simulink model "SP_Dynamic_17Okt_ExergyFlow"  (R2019b)
settings: Solver=FixedStepAuto  StartTime=0.0  StopTime=0  FixedStep=1/3600  RelTol=1e-3
model workspace (MAT data in the model file):
  AD : Simulink.Parameter (value not decoded)
  AG : Simulink.Parameter (value not decoded)
  AH : Simulink.Parameter (value not decoded)
  AV : Simulink.Parameter (value not decoded)
  AVP : Simulink.Parameter (value not decoded)
  BCHL : Simulink.Parameter (value not decoded)
  BCHV : Simulink.Parameter (value not decoded)
  BD : Simulink.Parameter (value not decoded)
  BG : Simulink.Parameter (value not decoded)
  BH : Simulink.Parameter (value not decoded)
  BVP : Simulink.Parameter (value not decoded)
  CD : Simulink.Parameter (value not decoded)
  CG : Simulink.Parameter (value not decoded)
  CH : Simulink.Parameter (value not decoded)
  CVP : Simulink.Parameter (value not decoded)
  XMW : Simulink.Parameter (value not decoded)
symbols that are objects in the model workspace (value not decoded): AD, AG, AH, AV, AVP, BD, BG, BH, BVP, CD, CG, CH, CVP, XMW
undefined symbols (not defined in the file or in its folder): magnitude, SETPT, XMEAS, XMV
libraries: mylib x165, dspindex x17
(part 10 of 10)

== system SP_Dynamic_17Okt_ExergyFlow/Random number generator/Process Measurements XMEAS(I) I=1-22/If Action Subsystem3/Subsystem/Subsystem2/TESUB6 XMNS(12) ==
  G : Inport
  Process Noise I=1-12 G New : mylib/Process Noise I=1-12 G New  SystemSampleTime=-1  Latency=0  AutoFrameSizeCalculation=off
  XNS(12) : Constant  Value=1.0000
  XMNS : Outport  VectorParamsAs1DForOutWhenUnconnected=off
  G_NEW : Outport  Port=2  VectorParamsAs1DForOutWhenUnconnected=off
  wires:
  XNS(12)/1 -> Process Noise I=1-12 G New/1
  Process Noise I=1-12 G New/1 -> XMNS/1
  G/1 -> Process Noise I=1-12 G New/2
  Process Noise I=1-12 G New/2 -> G_NEW/1

== system SP_Dynamic_17Okt_ExergyFlow/Random number generator/Process Measurements XMEAS(I) I=1-22/If Action Subsystem3/Subsystem/Subsystem2/TESUB6 XMNS(13) ==
  G : Inport
  Process Noise I=1-12 G New : mylib/Process Noise I=1-12 G New  SystemSampleTime=-1  Latency=0  AutoFrameSizeCalculation=off
  XNS(13) : Constant  Value=0.3000
  XMNS : Outport  VectorParamsAs1DForOutWhenUnconnected=off
  G_NEW : Outport  Port=2  VectorParamsAs1DForOutWhenUnconnected=off
  wires:
  XNS(13)/1 -> Process Noise I=1-12 G New/1
  Process Noise I=1-12 G New/1 -> XMNS/1
  G/1 -> Process Noise I=1-12 G New/2
  Process Noise I=1-12 G New/2 -> G_NEW/1

== system SP_Dynamic_17Okt_ExergyFlow/Random number generator/Process Measurements XMEAS(I) I=1-22/If Action Subsystem3/Subsystem/Subsystem2/TESUB6 XMNS(14) ==
  G : Inport
  Process Noise I=1-12 G New : mylib/Process Noise I=1-12 G New  SystemSampleTime=-1  Latency=0  AutoFrameSizeCalculation=off
  XNS(14) : Constant  Value=0.1250
  XMNS : Outport  VectorParamsAs1DForOutWhenUnconnected=off
  G_NEW : Outport  Port=2  VectorParamsAs1DForOutWhenUnconnected=off
  wires:
  XNS(14)/1 -> Process Noise I=1-12 G New/1
  Process Noise I=1-12 G New/1 -> XMNS/1
  G/1 -> Process Noise I=1-12 G New/2
  Process Noise I=1-12 G New/2 -> G_NEW/1

== system SP_Dynamic_17Okt_ExergyFlow/Random number generator/Process Measurements XMEAS(I) I=1-22/If Action Subsystem3/Subsystem/Subsystem2/TESUB6 XMNS(15) ==
  G : Inport
  Process Noise I=1-12 G New : mylib/Process Noise I=1-12 G New  SystemSampleTime=-1  Latency=0  AutoFrameSizeCalculation=off
  XNS(15) : Constant  Value=1.0000
  XMNS : Outport  VectorParamsAs1DForOutWhenUnconnected=off
  G_NEW : Outport  Port=2  VectorParamsAs1DForOutWhenUnconnected=off
  wires:
  XNS(15)/1 -> Process Noise I=1-12 G New/1
  Process Noise I=1-12 G New/1 -> XMNS/1
  G/1 -> Process Noise I=1-12 G New/2
  Process Noise I=1-12 G New/2 -> G_NEW/1

== system SP_Dynamic_17Okt_ExergyFlow/Random number generator/Process Measurements XMEAS(I) I=1-22/If Action Subsystem3/Subsystem/Subsystem3/TESUB6 XMNS(16) ==
  G : Inport
  Process Noise I=1-12 G New : mylib/Process Noise I=1-12 G New  SystemSampleTime=-1  Latency=0  AutoFrameSizeCalculation=off
  XNS(16) : Constant  Value=0.3000
  XMNS : Outport  VectorParamsAs1DForOutWhenUnconnected=off
  G_NEW : Outport  Port=2  VectorParamsAs1DForOutWhenUnconnected=off
  wires:
  XNS(16)/1 -> Process Noise I=1-12 G New/1
  Process Noise I=1-12 G New/1 -> XMNS/1
  G/1 -> Process Noise I=1-12 G New/2
  Process Noise I=1-12 G New/2 -> G_NEW/1

== system SP_Dynamic_17Okt_ExergyFlow/Random number generator/Process Measurements XMEAS(I) I=1-22/If Action Subsystem3/Subsystem/Subsystem3/TESUB6 XMNS(17) ==
  G : Inport
  Process Noise I=1-12 G New : mylib/Process Noise I=1-12 G New  SystemSampleTime=-1  Latency=0  AutoFrameSizeCalculation=off
  XNS(17) : Constant  Value=0.1150
  XMNS : Outport  VectorParamsAs1DForOutWhenUnconnected=off
  G_NEW : Outport  Port=2  VectorParamsAs1DForOutWhenUnconnected=off
  wires:
  XNS(17)/1 -> Process Noise I=1-12 G New/1
  Process Noise I=1-12 G New/1 -> XMNS/1
  G/1 -> Process Noise I=1-12 G New/2
  Process Noise I=1-12 G New/2 -> G_NEW/1

== system SP_Dynamic_17Okt_ExergyFlow/Random number generator/Process Measurements XMEAS(I) I=1-22/If Action Subsystem3/Subsystem/Subsystem3/TESUB6 XMNS(18) ==
  G : Inport
  Process Noise I=1-12 G New : mylib/Process Noise I=1-12 G New  SystemSampleTime=-1  Latency=0  AutoFrameSizeCalculation=off
  XNS(18) : Constant  Value=0.0100
  XMNS : Outport  VectorParamsAs1DForOutWhenUnconnected=off
  G_NEW : Outport  Port=2  VectorParamsAs1DForOutWhenUnconnected=off
  wires:
  XNS(18)/1 -> Process Noise I=1-12 G New/1
  Process Noise I=1-12 G New/1 -> XMNS/1
  G/1 -> Process Noise I=1-12 G New/2
  Process Noise I=1-12 G New/2 -> G_NEW/1

== system SP_Dynamic_17Okt_ExergyFlow/Random number generator/Process Measurements XMEAS(I) I=1-22/If Action Subsystem3/Subsystem/Subsystem3/TESUB6 XMNS(19) ==
  G : Inport
  Process Noise I=1-12 G New : mylib/Process Noise I=1-12 G New  SystemSampleTime=-1  Latency=0  AutoFrameSizeCalculation=off
  XNS(19) : Constant  Value=1.1500
  XMNS : Outport  VectorParamsAs1DForOutWhenUnconnected=off
  G_NEW : Outport  Port=2  VectorParamsAs1DForOutWhenUnconnected=off
  wires:
  XNS(19)/1 -> Process Noise I=1-12 G New/1
  Process Noise I=1-12 G New/1 -> XMNS/1
  G/1 -> Process Noise I=1-12 G New/2
  Process Noise I=1-12 G New/2 -> G_NEW/1

== system SP_Dynamic_17Okt_ExergyFlow/Random number generator/Process Measurements XMEAS(I) I=1-22/If Action Subsystem3/Subsystem/Subsystem3/TESUB6 XMNS(20) ==
  G : Inport
  Process Noise I=1-12 G New : mylib/Process Noise I=1-12 G New  SystemSampleTime=-1  Latency=0  AutoFrameSizeCalculation=off
  XNS(20) : Constant  Value=0.2000
  XMNS : Outport  VectorParamsAs1DForOutWhenUnconnected=off
  G_NEW : Outport  Port=2  VectorParamsAs1DForOutWhenUnconnected=off
  wires:
  XNS(20)/1 -> Process Noise I=1-12 G New/1
  Process Noise I=1-12 G New/1 -> XMNS/1
  G/1 -> Process Noise I=1-12 G New/2
  Process Noise I=1-12 G New/2 -> G_NEW/1

== system SP_Dynamic_17Okt_ExergyFlow/Random number generator/Process Measurements XMEAS(I) I=1-22/If Action Subsystem3/Subsystem/Subsystem3/TESUB6 XMNS(21) ==
  G : Inport
  Process Noise I=1-12 G New : mylib/Process Noise I=1-12 G New  SystemSampleTime=-1  Latency=0  AutoFrameSizeCalculation=off
  XNS(21) : Constant  Value=0.0100
  XMNS : Outport  VectorParamsAs1DForOutWhenUnconnected=off
  G_NEW : Outport  Port=2  VectorParamsAs1DForOutWhenUnconnected=off
  wires:
  XNS(21)/1 -> Process Noise I=1-12 G New/1
  Process Noise I=1-12 G New/1 -> XMNS/1
  G/1 -> Process Noise I=1-12 G New/2
  Process Noise I=1-12 G New/2 -> G_NEW/1

== system SP_Dynamic_17Okt_ExergyFlow/Random number generator/Process Measurements XMEAS(I) I=1-22/If Action Subsystem3/Subsystem/Subsystem3/TESUB6 XMNS(22) ==
  G : Inport
  Process Noise I=1-12 G New : mylib/Process Noise I=1-12 G New  SystemSampleTime=-1  Latency=0  AutoFrameSizeCalculation=off
  XNS(22) : Constant  Value=0.0100
  XMNS : Outport  VectorParamsAs1DForOutWhenUnconnected=off
  G_NEW : Outport  Port=2  VectorParamsAs1DForOutWhenUnconnected=off
  wires:
  XNS(22)/1 -> Process Noise I=1-12 G New/1
  Process Noise I=1-12 G New/1 -> XMNS/1
  G/1 -> Process Noise I=1-12 G New/2
  Process Noise I=1-12 G New/2 -> G_NEW/1

== system SP_Dynamic_17Okt_ExergyFlow/Random number generator/Process Measurements XMEAS(I) I=23-36/If Action Subsystem3/Subsystem/Subsystem/TESUB6 XMNS(23) ==
  G : Inport
  Process Noise I=1-12 G New : mylib/Process Noise I=1-12 G New  SystemSampleTime=-1  Latency=0  AutoFrameSizeCalculation=off
  XNS(23) : Constant  Value=0.25
  XMNS : Outport  VectorParamsAs1DForOutWhenUnconnected=off
  G_NEW : Outport  Port=2  VectorParamsAs1DForOutWhenUnconnected=off
  wires:
  XNS(23)/1 -> Process Noise I=1-12 G New/1
  Process Noise I=1-12 G New/1 -> XMNS/1
  G/1 -> Process Noise I=1-12 G New/2
  Process Noise I=1-12 G New/2 -> G_NEW/1

== system SP_Dynamic_17Okt_ExergyFlow/Random number generator/Process Measurements XMEAS(I) I=23-36/If Action Subsystem3/Subsystem/Subsystem/TESUB6 XMNS(24) ==
  G : Inport
  Process Noise I=1-12 G New : mylib/Process Noise I=1-12 G New  SystemSampleTime=-1  Latency=0  AutoFrameSizeCalculation=off
  XNS(24) : Constant  Value=0.1
  XMNS : Outport  VectorParamsAs1DForOutWhenUnconnected=off
  G_NEW : Outport  Port=2  VectorParamsAs1DForOutWhenUnconnected=off
  wires:
  XNS(24)/1 -> Process Noise I=1-12 G New/1
  Process Noise I=1-12 G New/1 -> XMNS/1
  G/1 -> Process Noise I=1-12 G New/2
  Process Noise I=1-12 G New/2 -> G_NEW/1

== system SP_Dynamic_17Okt_ExergyFlow/Random number generator/Process Measurements XMEAS(I) I=23-36/If Action Subsystem3/Subsystem/Subsystem/TESUB6 XMNS(25) ==
  G : Inport
  Process Noise I=1-12 G New : mylib/Process Noise I=1-12 G New  SystemSampleTime=-1  Latency=0  AutoFrameSizeCalculation=off
  XNS(25) : Constant  Value=0.25
  XMNS : Outport  VectorParamsAs1DForOutWhenUnconnected=off
  G_NEW : Outport  Port=2  VectorParamsAs1DForOutWhenUnconnected=off
  wires:
  XNS(25)/1 -> Process Noise I=1-12 G New/1
  Process Noise I=1-12 G New/1 -> XMNS/1
  G/1 -> Process Noise I=1-12 G New/2
  Process Noise I=1-12 G New/2 -> G_NEW/1

== system SP_Dynamic_17Okt_ExergyFlow/Random number generator/Process Measurements XMEAS(I) I=23-36/If Action Subsystem3/Subsystem/Subsystem/TESUB6 XMNS(26) ==
  G : Inport
  Process Noise I=1-12 G New : mylib/Process Noise I=1-12 G New  SystemSampleTime=-1  Latency=0  AutoFrameSizeCalculation=off
  XNS(26) : Constant  Value=0.1
  XMNS : Outport  VectorParamsAs1DForOutWhenUnconnected=off
  G_NEW : Outport  Port=2  VectorParamsAs1DForOutWhenUnconnected=off
  wires:
  XNS(26)/1 -> Process Noise I=1-12 G New/1
  Process Noise I=1-12 G New/1 -> XMNS/1
  G/1 -> Process Noise I=1-12 G New/2
  Process Noise I=1-12 G New/2 -> G_NEW/1

== system SP_Dynamic_17Okt_ExergyFlow/Random number generator/Process Measurements XMEAS(I) I=23-36/If Action Subsystem3/Subsystem/Subsystem/TESUB6 XMNS(27) ==
  G : Inport
  Process Noise I=1-12 G New : mylib/Process Noise I=1-12 G New  SystemSampleTime=-1  Latency=0  AutoFrameSizeCalculation=off
  XNS(27) : Constant  Value=0.25
  XMNS : Outport  VectorParamsAs1DForOutWhenUnconnected=off
  G_NEW : Outport  Port=2  VectorParamsAs1DForOutWhenUnconnected=off
  wires:
  XNS(27)/1 -> Process Noise I=1-12 G New/1
  Process Noise I=1-12 G New/1 -> XMNS/1
  G/1 -> Process Noise I=1-12 G New/2
  Process Noise I=1-12 G New/2 -> G_NEW/1

== system SP_Dynamic_17Okt_ExergyFlow/Random number generator/Process Measurements XMEAS(I) I=23-36/If Action Subsystem3/Subsystem/Subsystem1/TESUB6 XMNS(28) ==
  G : Inport
  Process Noise I=1-12 G New : mylib/Process Noise I=1-12 G New  SystemSampleTime=-1  Latency=0  AutoFrameSizeCalculation=off
  XNS(28) : Constant  Value=0.025
  XMNS : Outport  VectorParamsAs1DForOutWhenUnconnected=off
  G_NEW : Outport  Port=2  VectorParamsAs1DForOutWhenUnconnected=off
  wires:
  XNS(28)/1 -> Process Noise I=1-12 G New/1
  Process Noise I=1-12 G New/1 -> XMNS/1
  G/1 -> Process Noise I=1-12 G New/2
  Process Noise I=1-12 G New/2 -> G_NEW/1

== system SP_Dynamic_17Okt_ExergyFlow/Random number generator/Process Measurements XMEAS(I) I=23-36/If Action Subsystem3/Subsystem/Subsystem1/TESUB6 XMNS(29) ==
  G : Inport
  Process Noise I=1-12 G New : mylib/Process Noise I=1-12 G New  SystemSampleTime=-1  Latency=0  AutoFrameSizeCalculation=off
  XNS(29) : Constant  Value=0.25
  XMNS : Outport  VectorParamsAs1DForOutWhenUnconnected=off
  G_NEW : Outport  Port=2  VectorParamsAs1DForOutWhenUnconnected=off
  wires:
  XNS(29)/1 -> Process Noise I=1-12 G New/1
  Process Noise I=1-12 G New/1 -> XMNS/1
  G/1 -> Process Noise I=1-12 G New/2
  Process Noise I=1-12 G New/2 -> G_NEW/1

== system SP_Dynamic_17Okt_ExergyFlow/Random number generator/Process Measurements XMEAS(I) I=23-36/If Action Subsystem3/Subsystem/Subsystem1/TESUB6 XMNS(30) ==
  G : Inport
  Process Noise I=1-12 G New : mylib/Process Noise I=1-12 G New  SystemSampleTime=-1  Latency=0  AutoFrameSizeCalculation=off
  XNS(30) : Constant  Value=0.1
  XMNS : Outport  VectorParamsAs1DForOutWhenUnconnected=off
  G_NEW : Outport  Port=2  VectorParamsAs1DForOutWhenUnconnected=off
  wires:
  XNS(30)/1 -> Process Noise I=1-12 G New/1
  Process Noise I=1-12 G New/1 -> XMNS/1
  G/1 -> Process Noise I=1-12 G New/2
  Process Noise I=1-12 G New/2 -> G_NEW/1

== system SP_Dynamic_17Okt_ExergyFlow/Random number generator/Process Measurements XMEAS(I) I=23-36/If Action Subsystem3/Subsystem/Subsystem1/TESUB6 XMNS(31) ==
  G : Inport
  Process Noise I=1-12 G New : mylib/Process Noise I=1-12 G New  SystemSampleTime=-1  Latency=0  AutoFrameSizeCalculation=off
  XNS(31) : Constant  Value=0.25
  XMNS : Outport  VectorParamsAs1DForOutWhenUnconnected=off
  G_NEW : Outport  Port=2  VectorParamsAs1DForOutWhenUnconnected=off
  wires:
  XNS(31)/1 -> Process Noise I=1-12 G New/1
  Process Noise I=1-12 G New/1 -> XMNS/1
  G/1 -> Process Noise I=1-12 G New/2
  Process Noise I=1-12 G New/2 -> G_NEW/1

== system SP_Dynamic_17Okt_ExergyFlow/Random number generator/Process Measurements XMEAS(I) I=23-36/If Action Subsystem3/Subsystem/Subsystem1/TESUB6 XMNS(32) ==
  G : Inport
  Process Noise I=1-12 G New : mylib/Process Noise I=1-12 G New  SystemSampleTime=-1  Latency=0  AutoFrameSizeCalculation=off
  XNS(32) : Constant  Value=0.1
  XMNS : Outport  VectorParamsAs1DForOutWhenUnconnected=off
  G_NEW : Outport  Port=2  VectorParamsAs1DForOutWhenUnconnected=off
  wires:
  XNS(32)/1 -> Process Noise I=1-12 G New/1
  Process Noise I=1-12 G New/1 -> XMNS/1
  G/1 -> Process Noise I=1-12 G New/2
  Process Noise I=1-12 G New/2 -> G_NEW/1

== system SP_Dynamic_17Okt_ExergyFlow/Random number generator/Process Measurements XMEAS(I) I=23-36/If Action Subsystem3/Subsystem/Subsystem2/TESUB6 XMNS(33) ==
  G : Inport
  Process Noise I=1-12 G New : mylib/Process Noise I=1-12 G New  SystemSampleTime=-1  Latency=0  AutoFrameSizeCalculation=off
  XNS(33) : Constant  Value=0.25
  XMNS : Outport  VectorParamsAs1DForOutWhenUnconnected=off
  G_NEW : Outport  Port=2  VectorParamsAs1DForOutWhenUnconnected=off
  wires:
  XNS(33)/1 -> Process Noise I=1-12 G New/1
  Process Noise I=1-12 G New/1 -> XMNS/1
  G/1 -> Process Noise I=1-12 G New/2
  Process Noise I=1-12 G New/2 -> G_NEW/1

== system SP_Dynamic_17Okt_ExergyFlow/Random number generator/Process Measurements XMEAS(I) I=23-36/If Action Subsystem3/Subsystem/Subsystem2/TESUB6 XMNS(34) ==
  G : Inport
  Process Noise I=1-12 G New : mylib/Process Noise I=1-12 G New  SystemSampleTime=-1  Latency=0  AutoFrameSizeCalculation=off
  XNS(34) : Constant  Value=0.025
  XMNS : Outport  VectorParamsAs1DForOutWhenUnconnected=off
  G_NEW : Outport  Port=2  VectorParamsAs1DForOutWhenUnconnected=off
  wires:
  XNS(34)/1 -> Process Noise I=1-12 G New/1
  Process Noise I=1-12 G New/1 -> XMNS/1
  G/1 -> Process Noise I=1-12 G New/2
  Process Noise I=1-12 G New/2 -> G_NEW/1

== system SP_Dynamic_17Okt_ExergyFlow/Random number generator/Process Measurements XMEAS(I) I=23-36/If Action Subsystem3/Subsystem/Subsystem2/TESUB6 XMNS(35) ==
  G : Inport
  Process Noise I=1-12 G New : mylib/Process Noise I=1-12 G New  SystemSampleTime=-1  Latency=0  AutoFrameSizeCalculation=off
  XNS(35) : Constant  Value=0.05
  XMNS : Outport  VectorParamsAs1DForOutWhenUnconnected=off
  G_NEW : Outport  Port=2  VectorParamsAs1DForOutWhenUnconnected=off
  wires:
  XNS(35)/1 -> Process Noise I=1-12 G New/1
  Process Noise I=1-12 G New/1 -> XMNS/1
  G/1 -> Process Noise I=1-12 G New/2
  Process Noise I=1-12 G New/2 -> G_NEW/1

== system SP_Dynamic_17Okt_ExergyFlow/Random number generator/Process Measurements XMEAS(I) I=23-36/If Action Subsystem3/Subsystem/Subsystem2/TESUB6 XMNS(36) ==
  G : Inport
  Process Noise I=1-12 G New : mylib/Process Noise I=1-12 G New  SystemSampleTime=-1  Latency=0  AutoFrameSizeCalculation=off
  XNS(36) : Constant  Value=0.05
  XMNS : Outport  VectorParamsAs1DForOutWhenUnconnected=off
  G_NEW : Outport  Port=2  VectorParamsAs1DForOutWhenUnconnected=off
  wires:
  XNS(36)/1 -> Process Noise I=1-12 G New/1
  Process Noise I=1-12 G New/1 -> XMNS/1
  G/1 -> Process Noise I=1-12 G New/2
  Process Noise I=1-12 G New/2 -> G_NEW/1

== system SP_Dynamic_17Okt_ExergyFlow/Random number generator/Process Measurements XMEAS(I) I=37-41/If Action Subsystem3/Subsystem/Subsystem/TESUB6 XMNS(37) ==
  G : Inport
  Process Noise I=1-12 G New : mylib/Process Noise I=1-12 G New  SystemSampleTime=-1  Latency=0  AutoFrameSizeCalculation=off
  XNS(37) : Constant  Value=0.01
  XMNS : Outport  VectorParamsAs1DForOutWhenUnconnected=off
  G_NEW : Outport  Port=2  VectorParamsAs1DForOutWhenUnconnected=off
  wires:
  XNS(37)/1 -> Process Noise I=1-12 G New/1
  Process Noise I=1-12 G New/1 -> XMNS/1
  G/1 -> Process Noise I=1-12 G New/2
  Process Noise I=1-12 G New/2 -> G_NEW/1

== system SP_Dynamic_17Okt_ExergyFlow/Random number generator/Process Measurements XMEAS(I) I=37-41/If Action Subsystem3/Subsystem/Subsystem/TESUB6 XMNS(38) ==
  G : Inport
  Process Noise I=1-12 G New : mylib/Process Noise I=1-12 G New  SystemSampleTime=-1  Latency=0  AutoFrameSizeCalculation=off
  XNS(38) : Constant  Value=0.01
  XMNS : Outport  VectorParamsAs1DForOutWhenUnconnected=off
  G_NEW : Outport  Port=2  VectorParamsAs1DForOutWhenUnconnected=off
  wires:
  XNS(38)/1 -> Process Noise I=1-12 G New/1
  Process Noise I=1-12 G New/1 -> XMNS/1
  G/1 -> Process Noise I=1-12 G New/2
  Process Noise I=1-12 G New/2 -> G_NEW/1

== system SP_Dynamic_17Okt_ExergyFlow/Random number generator/Process Measurements XMEAS(I) I=37-41/If Action Subsystem3/Subsystem/Subsystem/TESUB6 XMNS(39) ==
  G : Inport
  Process Noise I=1-12 G New : mylib/Process Noise I=1-12 G New  SystemSampleTime=-1  Latency=0  AutoFrameSizeCalculation=off
  XNS(39) : Constant  Value=0.01
  XMNS : Outport  VectorParamsAs1DForOutWhenUnconnected=off
  G_NEW : Outport  Port=2  VectorParamsAs1DForOutWhenUnconnected=off
  wires:
  XNS(39)/1 -> Process Noise I=1-12 G New/1
  Process Noise I=1-12 G New/1 -> XMNS/1
  G/1 -> Process Noise I=1-12 G New/2
  Process Noise I=1-12 G New/2 -> G_NEW/1

== system SP_Dynamic_17Okt_ExergyFlow/Random number generator/Process Measurements XMEAS(I) I=37-41/If Action Subsystem3/Subsystem/Subsystem/TESUB6 XMNS(40) ==
  G : Inport
  Process Noise I=1-12 G New : mylib/Process Noise I=1-12 G New  SystemSampleTime=-1  Latency=0  AutoFrameSizeCalculation=off
  XNS(40) : Constant  Value=0.5
  XMNS : Outport  VectorParamsAs1DForOutWhenUnconnected=off
  G_NEW : Outport  Port=2  VectorParamsAs1DForOutWhenUnconnected=off
  wires:
  XNS(40)/1 -> Process Noise I=1-12 G New/1
  Process Noise I=1-12 G New/1 -> XMNS/1
  G/1 -> Process Noise I=1-12 G New/2
  Process Noise I=1-12 G New/2 -> G_NEW/1

== system SP_Dynamic_17Okt_ExergyFlow/Random number generator/Process Measurements XMEAS(I) I=37-41/If Action Subsystem3/Subsystem/Subsystem/TESUB6 XMNS(41) ==
  G : Inport
  Process Noise I=1-12 G New : mylib/Process Noise I=1-12 G New  SystemSampleTime=-1  Latency=0  AutoFrameSizeCalculation=off
  XNS(41) : Constant  Value=0.5
  XMNS : Outport  VectorParamsAs1DForOutWhenUnconnected=off
  G_NEW : Outport  Port=2  VectorParamsAs1DForOutWhenUnconnected=off
  wires:
  XNS(41)/1 -> Process Noise I=1-12 G New/1
  Process Noise I=1-12 G New/1 -> XMNS/1
  G/1 -> Process Noise I=1-12 G New/2
  Process Noise I=1-12 G New/2 -> G_NEW/1

== system SP_Dynamic_17Okt_ExergyFlow/Subsystem/Braatz/ 10/CONTROL 6/P Control/ERR ==
  SETPT : Inport
  High Limit : Inport  Port=2
  XMEAS : Inport  Port=3
  " " : Product  Inputs=**/
  Bus Selector : BusSelector  OutputSignals=signal3.XMEAS(10)
  Constant : Constant  Value=100
  Subtract : Sum  Inputs=+-
  ERR : Outport  VectorParamsAs1DForOutWhenUnconnected=off
  wires:
  " "/1 -> ERR/1
  SETPT/1 -> Subtract/1
  Subtract/1 -> " "/1
  High Limit/1 -> " "/3
  Constant/1 -> " "/2
  XMEAS/1 -> Bus Selector/1
  Bus Selector/1 -> Subtract/2  "<XMEAS(10)>"

== system SP_Dynamic_17Okt_ExergyFlow/Subsystem/Braatz/ 10/CONTROL 6/P Control/Pressure limits ==
  "XMV(6) " : Inport
  XMEAS : Inport  Port=2
  Abs : Abs
  Bus Selector : BusSelector  OutputSignals=signal3.XMEAS(13)
  Constant : Constant  Value=100
  Constant1 : Constant  Value=0
  If : If  IfExpression=u1 >= 2950  ElseIfExpressions=u1 <= 2300
  If Action Subsystem : Subsystem  TreatAsAtomicUnit=on
  If Action Subsystem1 : Subsystem  TreatAsAtomicUnit=on
  If Action Subsystem2 : Subsystem  TreatAsAtomicUnit=on
  Merge : Merge  Inputs=3
  Subsystem1 : mylib/Braatz Control/Subsystem1  SystemSampleTime=-1  Latency=0  AutoFrameSizeCalculation=off
  XMV(6) : Outport  VectorParamsAs1DForOutWhenUnconnected=off
  wires:
  If/1 -> If Action Subsystem/Action
  Constant1/1 -> If Action Subsystem1/1(In1)
  Merge/1 -> Abs/1
  If/3 -> If Action Subsystem2/Action
  Constant/1 -> If Action Subsystem/1(In1)
  Bus Selector/1 -> If/1  "<XMEAS(13)>"
  If Action Subsystem2/1(Out1) -> Merge/3
  If Action Subsystem1/1(Out1) -> Merge/2
  XMEAS/1 -> Bus Selector/1
  If/2 -> If Action Subsystem1/Action
  If Action Subsystem/1(Out1) -> Merge/1
  "XMV(6) "/1 -> If Action Subsystem2/1(In1)
  Abs/1 -> Subsystem1/1
  Subsystem1/1 -> XMV(6)/1

== system SP_Dynamic_17Okt_ExergyFlow/Subsystem/Braatz/ 10/CONTROL 6/P Control/Subsystem ==
  ERR : Inport
  GAIN : Inport  Port=2
  ERROLD : UnitDelay  SampleTime=-1  HasFrameUpgradeWarning=on
  Product : Product
  Subtract1 : Sum  Inputs=+-
  DXMV : Outport  VectorParamsAs1DForOutWhenUnconnected=off
  wires:
  ERR/1 -> Subtract1/1, ERROLD/1
  ERROLD/1 -> Subtract1/2
  Subtract1/1 -> Product/2
  Product/1 -> DXMV/1
  GAIN/1 -> Product/1

== system SP_Dynamic_17Okt_ExergyFlow/Subsystem/Braatz/ 10/CONTROL 6/P Control/Pressure limits/If Action Subsystem ==
  In1 : Inport
  Action Port : ActionPort  ActionPortLabel=if(u1 >= 2950)
  Out1 : Outport  VectorParamsAs1DForOutWhenUnconnected=off
  wires:
  In1/1 -> Out1/1

== system SP_Dynamic_17Okt_ExergyFlow/Subsystem/Braatz/ 10/CONTROL 6/P Control/Pressure limits/If Action Subsystem1 ==
  In1 : Inport
  Action Port : ActionPort  ActionPortLabel=elseif(u1 <= 2300)
  Out1 : Outport  VectorParamsAs1DForOutWhenUnconnected=off
  wires:
  In1/1 -> Out1/1

== system SP_Dynamic_17Okt_ExergyFlow/Subsystem/Braatz/ 10/CONTROL 6/P Control/Pressure limits/If Action Subsystem2 ==
  In1 : Inport
  Action Port : ActionPort  ActionPortLabel=else
  Out1 : Outport  VectorParamsAs1DForOutWhenUnconnected=off
  wires:
  In1/1 -> Out1/1

== matlab function SP_Dynamic_17Okt_ExergyFlow/Separator/TCS Initial Temperature in Separator °C /MATLAB Function ==
  data: AH input; TCS output; BH input; CH input; AG input; BG input; CG input; AV input; XMW input; XLS input; ETS input; UTLS input; ITY input; J output; TCS input
function [TCS,J] = TempLoop(AH,BH,CH,AG,BG,CG,AV,XMW,XLS,ETS,UTLS,ITY,TCS)

ESS = ETS/UTLS;
     
Z = XLS;
T = TCS;
H = ESS;
TIN=T;

for J = 1:100
	
	if ITY == 0
    	HTEST = 0;
		for I = 1:8
      		HI = T * (AH(I,1) + BH(I,1) * T / 2 + CH(I,1) * T^2 / 3);
      		HI = 1.8 * HI;
      		HTEST = HTEST + Z(I,1) * XMW(I,1) * HI;
		end
	else
      	HTEST = 0;
		for I = 1:8 
      		HI = T * (AG(I,1) + BG(I,1) * T / 2 + CG(I,1) * T^2 / 3);
      		HI = 1.8 * HI;
      		HI = HI + AV(I,1);
      		HTEST = HTEST + Z(I,1) * XMW(I,1) * HI;
		end
    end
        if ITY == 2
         	R1 = 3.57696 / 1000000;
        	HTEST = HTEST - R1 * (T + 273.15);
    	end
		
    ERR = HTEST - H;
	
	if ITY == 0
      	DH = 0.0;
    	for I = 1:8
      		DHI = AH(I,1) + BH(I,1) * T + CH(I,1) * T^2;
      		DHI = 1.8 * DHI;
      		DH = DH + Z(I,1) * XMW(I,1) * DHI;
		end
	else
      	DH=0.0;
    	for I = 1:8
      		DHI = AG(I,1) + BG(I,1) * T + CG(I,1) * T^2;
      		DHI = 1.8 * DHI;
      		DH = DH + Z(I,1) * XMW(I,1) * DHI;
		end
    end
    
    if ITY == 2
      	R3 = 3.57696/1000000;
     	DH = DH - R3;
 	end
	
    DT = -ERR / DH;
    T = T + DT;
  	if abs(DT) < 1*10^(-12)
    	break
  	end
  	if J == 100
  		T = TIN;
  	end
end
TCS = T;

== matlab function SP_Dynamic_17Okt_ExergyFlow/Reactor/TCR Initial Temperature in Reactor °C /MATLAB Function ==
  data: AH input; TCR output; BH input; CH input; AG input; BG input; CG input; AV input; XMW input; XLR input; ETR input; UTLR input; ITY input; J output; TCR input
function [TCR,J] = TempLoop(AH,BH,CH,AG,BG,CG,AV,XMW,XLR,ETR,UTLR,ITY,TCR)

ESR = ETR/UTLR;
     
Z = XLR;
T = TCR;
H = ESR;
TIN=T;

for J = 1:100
	
	if ITY == 0
    	HTEST = 0;
		for I = 1:8
      		HI = T * (AH(I,1) + BH(I,1) * T / 2 + CH(I,1) * T^2 / 3);
      		HI = 1.8 * HI;
      		HTEST = HTEST + Z(I,1) * XMW(I,1) * HI;
		end
	else
      	HTEST = 0;
		for I = 1:8 
      		HI = T * (AG(I,1) + BG(I,1) * T / 2 + CG(I,1) * T^2 / 3);
      		HI = 1.8 * HI;
      		HI = HI + AV(I,1);
      		HTEST = HTEST + Z(I,1) * XMW(I,1) * HI;
		end
    end
        if ITY == 2
         	R1 = 3.57696 / 1000000;
        	HTEST = HTEST - R1 * (T + 273.15);
    	end
		
    ERR = HTEST - H;
	
	if ITY == 0
      	DH = 0.0;
    	for I = 1:8
      		DHI = AH(I,1) + BH(I,1) * T + CH(I,1) * T^2;
      		DHI = 1.8 * DHI;
      		DH = DH + Z(I,1) * XMW(I,1) * DHI;
		end
	else
      	DH=0.0;
    	for I = 1:8
      		DHI = AG(I,1) + BG(I,1) * T + CG(I,1) * T^2;
      		DHI = 1.8 * DHI;
      		DH = DH + Z(I,1) * XMW(I,1) * DHI;
		end
    end
    
    if ITY == 2
      	R3 = 3.57696/1000000;
     	DH = DH - R3;
 	end
	
    DT = -ERR / DH;
    T = T + DT;
  	if abs(DT) < 1*10^(-12)
    	break
  	end
  	if J == 100
  		T = TIN;
  	end
end
TCR = T;

== matlab function SP_Dynamic_17Okt_ExergyFlow/Stripper/TCC Initial Temperature in Stripper °C /MATLAB Function ==
  data: AH input; TCC output; BH input; CH input; AG input; BG input; CG input; AV input; XMW input; XLC input; ETC input; UTLC input; ITY input; J output; TCC input
function [TCC,J] = TempLoop(AH,BH,CH,AG,BG,CG,AV,XMW,XLC,ETC,UTLC,ITY,TCC)

ESC = ETC/UTLC;
     
Z = XLC;
T = TCC;
H = ESC;
TIN=T;

for J = 1:100
	
	if ITY == 0
    	HTEST = 0;
		for I = 1:8
      		HI = T * (AH(I,1) + BH(I,1) * T / 2 + CH(I,1) * T^2 / 3);
      		HI = 1.8 * HI;
      		HTEST = HTEST + Z(I,1) * XMW(I,1) * HI;
		end
	else
      	HTEST = 0;
		for I = 1:8 
      		HI = T * (AG(I,1) + BG(I,1) * T / 2 + CG(I,1) * T^2 / 3);
      		HI = 1.8 * HI;
      		HI = HI + AV(I,1);
      		HTEST = HTEST + Z(I,1) * XMW(I,1) * HI;
		end
    end
        if ITY == 2
         	R1 = 3.57696 / 1000000;
        	HTEST = HTEST - R1 * (T + 273.15);
    	end
		
    ERR = HTEST - H;
	
	if ITY == 0
      	DH = 0.0;
    	for I = 1:8
      		DHI = AH(I,1) + BH(I,1) * T + CH(I,1) * T^2;
      		DHI = 1.8 * DHI;
      		DH = DH + Z(I,1) * XMW(I,1) * DHI;
		end
	else
      	DH=0.0;
    	for I = 1:8
      		DHI = AG(I,1) + BG(I,1) * T + CG(I,1) * T^2;
      		DHI = 1.8 * DHI;
      		DH = DH + Z(I,1) * XMW(I,1) * DHI;
		end
    end
    
    if ITY == 2
      	R3 = 3.57696/1000000;
     	DH = DH - R3;
 	end
	
    DT = -ERR / DH;
    T = T + DT;
  	if abs(DT) < 1*10^(-12)
    	break
  	end
  	if J == 100
  		T = TIN;
  	end
end
TCC = T;

== matlab function SP_Dynamic_17Okt_ExergyFlow/Mixing Zone/TCV Initial Temperature in Mixing zone °C /MATLAB Function ==
  data: AH input; TCV output; BH input; CH input; AG input; BG input; CG input; AV input; XMW input; XVV input; ETV input; UTVV input; ITY input; J output; TCV input
function [TCV,J] = TempLoop(AH,BH,CH,AG,BG,CG,AV,XMW,XVV,ETV,UTVV,ITY,TCV)

ESV = ETV/UTVV;
     
Z = XVV;
T = TCV;
H = ESV;
TIN=T;

for J = 1:100
	
	if ITY == 0
    	HTEST = 0;
		for I = 1:8
      		HI = T * (AH(I,1) + BH(I,1) * T / 2 + CH(I,1) * T^2 / 3);
      		HI = 1.8 * HI;
      		HTEST = HTEST + Z(I,1) * XMW(I,1) * HI;
		end
	else
      	HTEST = 0;
		for I = 1:8 
      		HI = T * (AG(I,1) + BG(I,1) * T / 2 + CG(I,1) * T^2 / 3);
      		HI = 1.8 * HI;
      		HI = HI + AV(I,1);
      		HTEST = HTEST + Z(I,1) * XMW(I,1) * HI;
		end
    end
        if ITY == 2
         	R1 = 3.57696 / 1000000;
        	HTEST = HTEST - R1 * (T + 273.15);
    	end
		
    ERR = HTEST - H;
	
	if ITY == 0
      	DH = 0.0;
    	for I = 1:8
      		DHI = AH(I,1) + BH(I,1) * T + CH(I,1) * T^2;
      		DHI = 1.8 * DHI;
      		DH = DH + Z(I,1) * XMW(I,1) * DHI;
		end
	else
      	DH=0.0;
    	for I = 1:8
      		DHI = AG(I,1) + BG(I,1) * T + CG(I,1) * T^2;
      		DHI = 1.8 * DHI;
      		DH = DH + Z(I,1) * XMW(I,1) * DHI;
		end
    end
    
    if ITY == 2
      	R3 = 3.57696/1000000;
     	DH = DH - R3;
 	end
	
    DT = -ERR / DH;
    T = T + DT;
  	if abs(DT) < 1*10^(-12)
    	break
  	end
  	if J == 100
  		T = TIN;
  	end
end
TCV = T;
